simulink model "example_simulink"  (R2022a)
settings: Solver=FixedStepAuto  StartTime=0.0  StopTime=10  FixedStep=0.001  RelTol=1e-3
InitFcn:
  | params.Kp = 98.4128;
  | params.Ki = 0.4971;
  | params.Kd = 0-64.7658;
  | params.u_min = -10;
  | params.u_max =  10;
  | params.enable_anti_windup = true;
  | params.deriv_filter_hz = 1.3029/(2*pi);
  | 
  | pid_mex('init', params);
StopFcn:
  | pid_mex('reset');
libraries: simulink x6
settings Model: Creator=CVeSS  LastModifiedBy=CVeSS
settings DataIOCC: ReturnWorkspaceOutputs=off

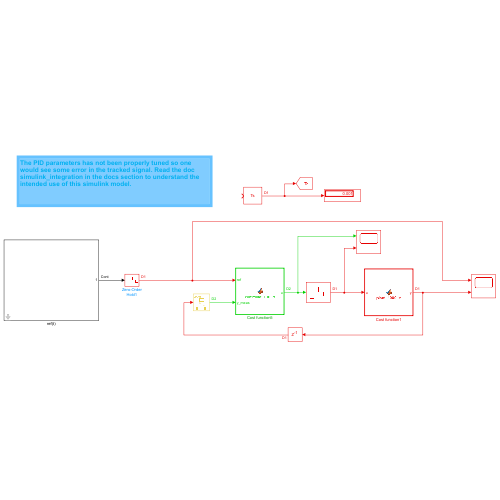
[thumbnail: Simulink's stored preview of the top-level diagram]
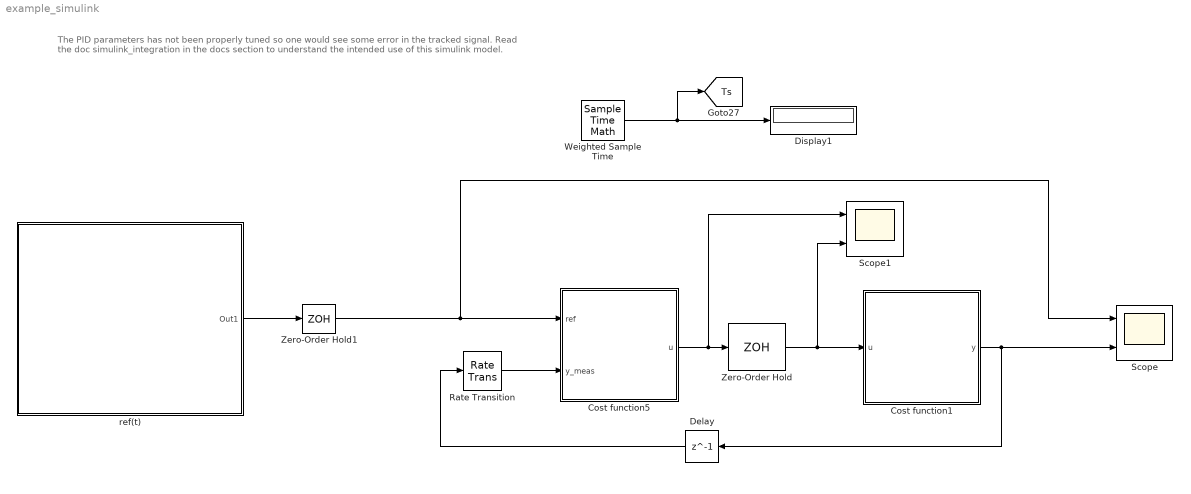
== system example_simulink ==
  note: The PID parameters has not been properly tuned so one would see some error in the tracked signal. Read the doc simulink_integration in the docs section to understand the intended use of this simulink model.
  Cost function1 : MATLAB Function  TreatAsAtomicUnit=on  SystemSampleTime=0.001
  Cost function5 : MATLAB Function  TreatAsAtomicUnit=on  SystemSampleTime=0.01
  Delay : Delay  DelayLength=1
  Display1 : Display
  Rate Transition : RateTransition  OutPortSampleTime=0.01
  Scope : Scope  NumInputPorts=2
  Scope1 : Scope  NumInputPorts=2
  Weighted Sample Time : SampleTimeMath  TsampMathOp=Ts Only
  Zero-Order Hold : ZeroOrderHold  SampleTime=0.001
  Zero-Order Hold1 : ZeroOrderHold  SampleTime=0.001
  ref(t) : Subsystem  mask{t_step_up=0.05, step_up_level=0.2, t_step_down=2, step_down_level=0.2, t_ramp_start=2, t_ramp_end=5, ramp_end_level=0.35, enable_wiggle=1, A_wiggle=0.05, f_wiggle=0.2, t_sine_start=5, t_sine_end=10, ref_min=0, ref_max=1.2}
      mask prompts: t_step_up "Step up time (s)"; step_up_level "Step up level"; t_step_down "Step down time (s)"; step_down_level "Step down level"; t_ramp_start "Ramp start time (s)"; t_ramp_end "Ramp end time (s)"; ramp_end_level "Ramp end level"; enable_wiggle "Enable wiggle (0 or 1)"; A_wiggle "Wiggle amplitude"; f_wiggle "Wiggle frequency (Hz)"; t_sine_start "sine start time (s)"; t_sine_end "sine end time (s)"
      mask DialogControl Container3 Prompt: Base reference (steps + ramps)
      mask DialogControl grpWiggle Prompt: Wiggle (small sine or chirp)
      mask DialogControl grpLimits Prompt: Reference limits
  tag scope: Ts=global
  wires:
  Weighted Sample Time/1 -> Display1/1, [Ts]
  Zero-Order Hold1/1 -> Scope/1, Cost function5/1(ref)
  Cost function5/1(u) -> Scope1/1, Zero-Order Hold/1
  Zero-Order Hold/1 -> Scope1/2, Cost function1/1(u)
  Cost function1/1(y) -> Delay/1, Scope/2
  Rate Transition/1 -> Cost function5/2(y_meas)
  Delay/1 -> Rate Transition/1
  ref(t)/1(Out1) -> Zero-Order Hold1/1

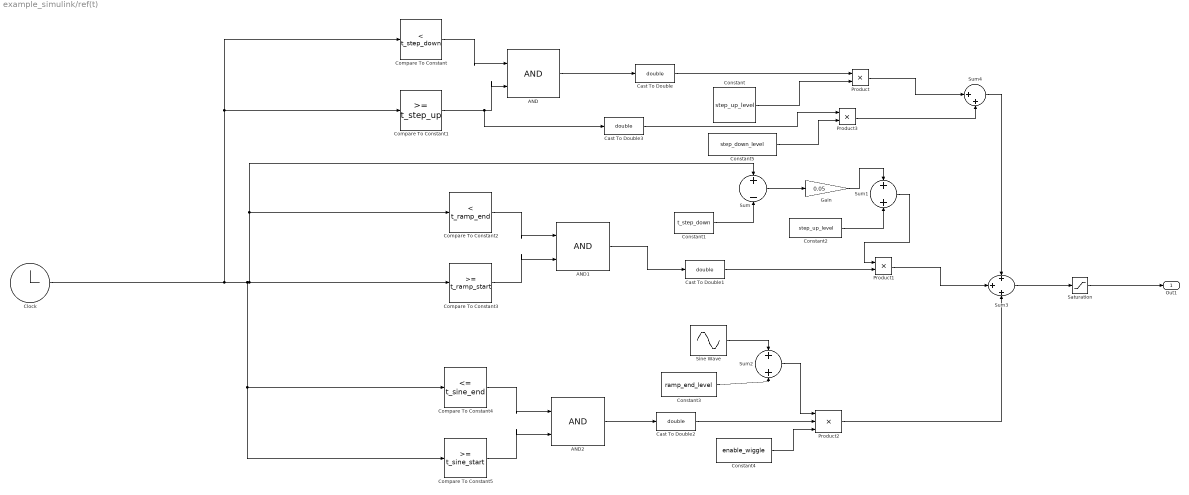
== system example_simulink/ref(t) ==
  AND : Logic  IconShape=distinctive  AllPortsSameDT=off  OutDataTypeStr=boolean
  AND1 : Logic  IconShape=distinctive  AllPortsSameDT=off  OutDataTypeStr=boolean
  AND2 : Logic  IconShape=distinctive  AllPortsSameDT=off  OutDataTypeStr=boolean
  Cast To Double{,1..3} (4 alike) : DataTypeConversion  OutDataTypeStr=double  SaturateOnIntegerOverflow=off  RndMeth=Floor
  Clock : Clock
  Compare To Constant : simulink/Logic and Bit Operations/Compare To Constant  relop=<  const=t_step_down  OutDataTypeStr=boolean
  Compare To Constant1 : simulink/Logic and Bit Operations/Compare To Constant  relop=>=  const=t_step_up  OutDataTypeStr=boolean
  Compare To Constant2 : simulink/Logic and Bit Operations/Compare To Constant  relop=<  const=t_ramp_end  OutDataTypeStr=boolean
  Compare To Constant3 : simulink/Logic and Bit Operations/Compare To Constant  relop=>=  const=t_ramp_start  OutDataTypeStr=boolean
  Compare To Constant4 : simulink/Logic and Bit Operations/Compare To Constant  relop=<=  const=t_sine_end  OutDataTypeStr=boolean
  Compare To Constant5 : simulink/Logic and Bit Operations/Compare To Constant  relop=>=  const=t_sine_start  OutDataTypeStr=boolean
  Constant : Constant  Value=step_up_level
  Constant1 : Constant  Value=t_step_down
  Constant2 : Constant  Value=step_up_level
  Constant3 : Constant  Value=ramp_end_level
  Constant4 : Constant  Value=enable_wiggle
  Constant5 : Constant  Value=step_down_level
  Gain : Gain  Gain=0.05
  Product : Product
  Product1 : Product
  Product2 : Product  Inputs=3
  Product3 : Product
  Saturation : Saturate  UpperLimit=ref_max  LowerLimit=ref_min
  Sine Wave : Sin  Amplitude=A_wiggle  Frequency=2*pi*f_wiggle  SampleTime=0
  Sum : Sum  Inputs=+-
  Sum1 : Sum
  Sum2 : Sum
  Sum3 : Sum  Inputs=+++
  Sum4 : Sum  Inputs=|++
  Out1 : Outport
  wires:
  Compare To Constant1/1 -> Cast To Double3/1, AND/2
  Compare To Constant2/1 -> AND1/1
  Constant2/1 -> Sum1/2
  Compare To Constant3/1 -> AND1/2
  AND1/1 -> Cast To Double1/1
  Product2/1 -> Sum3/3
  Sum1/1 -> Product1/1
  Clock/1 -> Compare To Constant5/1, Compare To Constant4/1, Sum/1, Compare To Constant2/1, Compare To Constant3/1, Compare To Constant/1, Compare To Constant1/1
  Sum/1 -> Gain/1
  Sum3/1 -> Saturation/1
  Constant/1 -> Product/2
  Gain/1 -> Sum1/1
  AND/1 -> Cast To Double/1
  Product1/1 -> Sum3/2
  Compare To Constant/1 -> AND/1
  Cast To Double1/1 -> Product1/2
  Constant1/1 -> Sum/2
  Cast To Double2/1 -> Product2/2
  Sum2/1 -> Product2/1
  Sine Wave/1 -> Sum2/1
  Compare To Constant4/1 -> AND2/1
  AND2/1 -> Cast To Double2/1
  Compare To Constant5/1 -> AND2/2
  Product/1 -> Sum4/1
  Cast To Double/1 -> Product/1
  Constant3/1 -> Sum2/2
  Saturation/1 -> Out1/1
  Constant4/1 -> Product2/3
  Cast To Double3/1 -> Product3/1
  Constant5/1 -> Product3/2
  Sum4/1 -> Sum3/1
  Product3/1 -> Sum4/2

== matlab function example_simulink/Cost function1 ==
  data: u input; y output
function y = plant_1000Hz(u)
persistent yk
if isempty(yk)
    yk = 0;
end

Ts = 0.001;
tau = 0.3;
K = 1.0;

a = exp(-Ts/tau);
b = (1 - a)*K;

yk = a*yk + b*u;
y = yk;
end

== matlab function example_simulink/Cost function5 ==
  data: ref input; u output; y_meas input
function u = controller_100Hz(ref, y_meas)
% Call MEX from MATLAB execution (not codegen)

coder.extrinsic('pid_mex');

dt_ctrl = 0.01;

% Pre-allocate output as a double so Simulink knows the type/size
u = 0.0;

% Call MEX. This executes in MATLAB, not generated code.
u = pid_mex('step', ref, y_meas, dt_ctrl);
end
